simulink model "Control_System"  (R2018b)
settings: Solver=FixedStepAuto  StartTime=0.0  StopTime=10.0  FixedStep=global_time_step  RelTol=1e-3
values from neighbouring files (symbols this model uses):
  SRC_Ts = global_time_step    (= 0.001)    [Parameters.m]
  TFO_Ts = global_time_step    (= 0.001)    [Parameters.m]
undefined symbols (not defined in the file or in its folder): DiscIntNeverNeededParam, tyre_radius
libraries: simulink x2
settings Model: PauseTimes=1  Creator=univ4123  LastModifiedBy=univ4123
settings OptimizationCC: LifeSpan=inf
settings DebuggingCC: SFUnexpectedBacktrackingDiag=warning  SFNoUnconditionalDefaultTransitionDiag=warning
settings SFSimCC: SimUseLocalCustomCode=off
settings RTWCC: GenCodeOnly=on  RTWUseLocalCustomCode=off  Toolchain=MinGW64 | gmake (64-bit Windows)
settings CodeAppCC: StateflowObjectComments=on
settings GRTTargetCC: GeneratePreprocessorConditionals=Disable all
settings ConfigComp: CovMetricSettings=dw  CovHtmlReporting=on  CovSaveCumulativeToWorkspaceVar=on  CovSaveSingleToWorkspaceVar=on  CovExternalEMLEnable=off

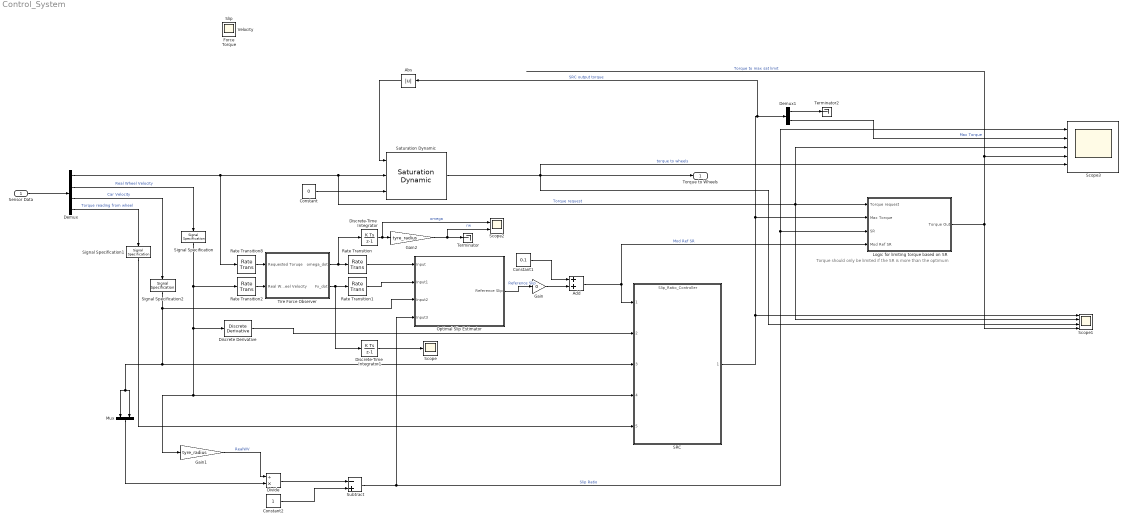
== system Control_System ==
  note: Torque should only be limited if the SR is more than the optimum
  Sensor Data : Inport
  Abs : Abs
  Add : Sum
  Constant : Constant  Value=0
  Constant1 : Constant  Value=0.1  SampleTime=SRC_Ts
  Constant2 : Constant  SampleTime=SRC_Ts
  Demux : Demux
  Demux1 : Demux  Outputs=2
  Discrete Derivative : simulink/Discrete/Discrete Derivative  gainval=1.0  ICPrevScaledInput=0.0  OutMin=[]  OutMax=[]  OutDataType=fixdt(1, 16)  OutScaling=2^-10  DoSatur=off
  Discrete-Time Integrator : DiscreteIntegrator  SampleTime=TFO_Ts  ICPrevOutput=DiscIntNeverNeededParam  ICPrevScaledInput=DiscIntNeverNeededParam
  Discrete-Time Integrator1 : DiscreteIntegrator  SampleTime=-1  ICPrevOutput=DiscIntNeverNeededParam  ICPrevScaledInput=DiscIntNeverNeededParam
  Divide : Product  Inputs=/*
  Gain : Gain  Gain=0
  Gain1 : Gain  Gain=tyre_radius
  Gain2 : Gain  Gain=tyre_radius
  Logic for limiting torque based on SR : Subsystem
  Mux : Mux  Inputs=2
  Optimal Slip Estimator : Subsystem
  Rate Transition : RateTransition  OutPortSampleTime=OSE_Ts
  Rate Transition1 : RateTransition  OutPortSampleTime=OSE_Ts
  Rate Transition2 : RateTransition  OutPortSampleTime=TFO_Ts
  Rate Transition8 : RateTransition  OutPortSampleTime=TFO_Ts
  SRC : ModelReference  ModelNameDialog=Slip_Ratio_Controller.slx  SimulationMode=Normal  ModelReferenceVersion=1.104
  Saturation Dynamic : simulink/Discontinuities/Saturation Dynamic  OutMin=[]  OutMax=[]  OutDataTypeStr=Inherit: Same as second input  OutDataType=fixdt(1, 16)  OutScaling=2^-10  DoSatur=off
  Scope : Scope
  Scope1 : Scope  NumInputPorts=4
  Scope2 : Scope  NumInputPorts=2
  Scope3 : Scope  NumInputPorts=5
  Signal Specification : SignalSpecification  Dimensions=[2 1]
  Signal Specification1 : SignalSpecification  Dimensions=1
  Signal Specification2 : SignalSpecification  Dimensions=1
  Subtract : Sum  Inputs=-+
  Terminator : Terminator
  Terminator2 : Terminator
  Tire Force Observer : Subsystem
  Torque to Wheels : Outport
  Force : Scope
  Slip : Scope
  Torque : Scope
  Velocity : Scope
  wires:
  Demux/1 -> Scope1/2, Scope3/3, Logic for limiting torque based on SR/1(Torque request), Saturation Dynamic/2, Rate Transition8/1  "Torque request"
  Saturation Dynamic/1 -> Scope1/3, Torque to Wheels/1, Scope3/5  "torque to wheels"
  Tire Force Observer/1(omega_dot) -> Discrete-Time Integrator/1, Rate Transition/1
  SRC/1 -> Abs/1, Demux1/1, Logic for limiting torque based on SR/2(Max Torque), Scope1/1  "SRC output torque"
  Constant/1 -> Saturation Dynamic/3
  Sensor Data/1 -> Demux/1
  Demux/2 -> Signal Specification/1  "Real Wheel Velocity"
  Demux/3 -> Signal Specification2/1  "Car Velocity"
  Rate Transition/1 -> Optimal Slip Estimator/1(Input)
  Tire Force Observer/2(Fx_dot) -> Discrete-Time Integrator1/1, Rate Transition1/1
  Gain/1 -> Add/2
  Constant1/1 -> Add/1
  Discrete-Time Integrator/1 -> Scope2/1, Gain2/1  "omega"
  Demux/4 -> Signal Specification1/1  "Torque reading from wheel"
  Rate Transition8/1 -> Tire Force Observer/1(Requested Toruqe)
  Rate Transition2/1 -> Tire Force Observer/2(Real Wheel Velocity)
  Rate Transition1/1 -> Optimal Slip Estimator/2(Input1)
  Signal Specification1/1 -> SRC/5
  Signal Specification2/1 -> Optimal Slip Estimator/3(Input2), Mux/1, Mux/2, SRC/3
  Logic for limiting torque based on SR/1(Torque Out) -> Scope3/4, Scope1/4  "Torque to max sat limit"
  Signal Specification/1 -> Rate Transition2/1, Gain1/1, SRC/4, Discrete Derivative/1
  Divide/1 -> Subtract/1
  Mux/1 -> Divide/2
  Gain1/1 -> Divide/1  "RealWV"
  Constant2/1 -> Subtract/2
  Add/1 -> Logic for limiting torque based on SR/4(Mod Ref SR), SRC/1  "Mod Ref SR"
  Optimal Slip Estimator/1(Reference Slip) -> Gain/1  "Reference Slip"
  Gain2/1 -> Scope2/2, Terminator/1  "rw"
  Discrete-Time Integrator1/1 -> Scope/1
  Discrete Derivative/1 -> SRC/2
  Subtract/1 -> Optimal Slip Estimator/4(Input3), Scope3/1, Logic for limiting torque based on SR/3(SR)  "Slip Ratio"
  Demux1/2 -> Scope3/2  "Max Torque"
  Demux1/1 -> Terminator2/1
  Abs/1 -> Saturation Dynamic/1

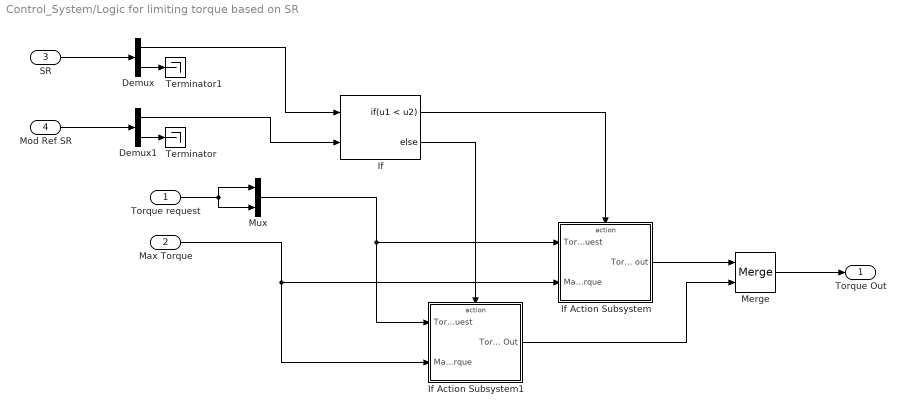
== system Control_System/Logic for limiting torque based on SR ==
  Torque request : Inport
  Max Torque : Inport  Port=2
  SR : Inport  Port=3
  Mod Ref SR : Inport  Port=4
  Demux : Demux  Outputs=2
  Demux1 : Demux  Outputs=2
  If : If  NumInputs=2  IfExpression=u1 < u2
  If Action Subsystem : Subsystem  TreatAsAtomicUnit=on
  If Action Subsystem1 : Subsystem  TreatAsAtomicUnit=on
  Merge : Merge
  Mux : Mux  Inputs=2
  Terminator : Terminator
  Terminator1 : Terminator
  Torque Out : Outport
  wires:
  SR/1 -> Demux/1
  Mod Ref SR/1 -> Demux1/1
  If/2 -> If Action Subsystem1/Action
  Mux/1 -> If Action Subsystem1/1(Torque Request), If Action Subsystem/1(Torque Request)
  Max Torque/1 -> If Action Subsystem1/2(Max Torque), If Action Subsystem/2(Max Torque)
  Merge/1 -> Torque Out/1
  If Action Subsystem/1(Torque out) -> Merge/1
  If Action Subsystem1/1(Torque Out) -> Merge/2
  Demux/1 -> If/1
  If/1 -> If Action Subsystem/Action
  Torque request/1 -> Mux/2, Mux/1
  Demux1/1 -> If/2
  Demux1/2 -> Terminator/1
  Demux/2 -> Terminator1/1

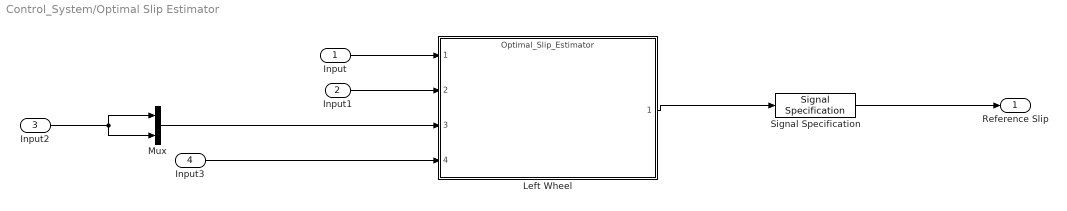
== system Control_System/Optimal Slip Estimator ==
  Input : Inport
  Input1 : Inport  Port=2
  Input2 : Inport  Port=3
  Input3 : Inport  Port=4
  Left Wheel : ModelReference  ModelNameDialog=Optimal_Slip_Estimator  SimulationMode=Normal  ModelReferenceVersion=1.13
  Mux : Mux  Inputs=2
  Signal Specification : SignalSpecification  Dimensions=[2 1]
  Reference Slip : Outport
  wires:
  Left Wheel/1 -> Signal Specification/1
  Signal Specification/1 -> Reference Slip/1
  Input/1 -> Left Wheel/1
  Input1/1 -> Left Wheel/2
  Input3/1 -> Left Wheel/4
  Mux/1 -> Left Wheel/3
  Input2/1 -> Mux/2, Mux/1

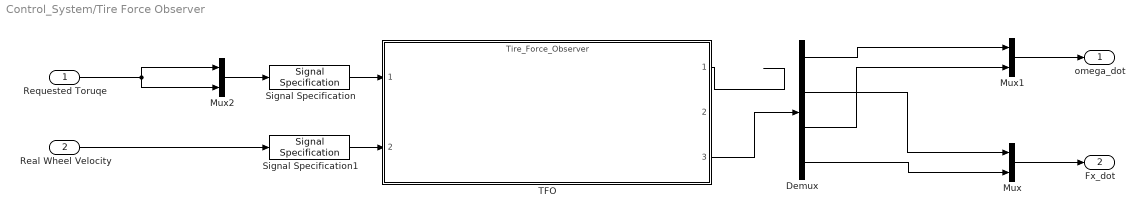
== system Control_System/Tire Force Observer ==
  Requested Toruqe : Inport
  Real Wheel Velocity : Inport  Port=2
  Demux : Demux
  Mux : Mux  Inputs=2
  Mux1 : Mux  Inputs=2
  Mux2 : Mux  Inputs=2
  Signal Specification : SignalSpecification  Dimensions=[2 1]
  Signal Specification1 : SignalSpecification  Dimensions=[2 1]
  TFO : ModelReference  ModelNameDialog=Tire_Force_Observer.slx  SimulationMode=Normal  ModelReferenceVersion=1.6
  omega_dot : Outport
  Fx_dot : Outport  Port=2
  wires:
  Requested Toruqe/1 -> Mux2/2, Mux2/1
  Real Wheel Velocity/1 -> Signal Specification1/1
  TFO/1 -> ?
  Mux1/1 -> omega_dot/1
  Demux/4 -> Mux/2
  Mux/1 -> Fx_dot/1
  Demux/2 -> Mux/1
  Demux/3 -> Mux1/2
  Demux/1 -> Mux1/1
  Mux2/1 -> Signal Specification/1
  Signal Specification/1 -> TFO/1
  Signal Specification1/1 -> TFO/2
  TFO/3 -> Demux/1

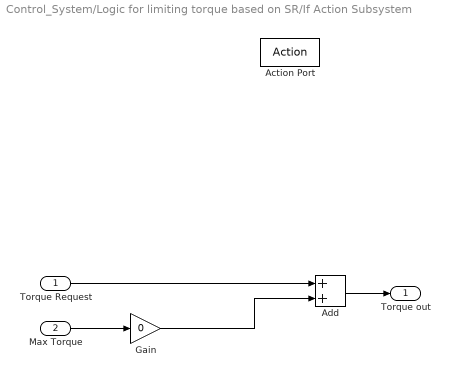
== system Control_System/Logic for limiting torque based on SR/If Action Subsystem ==
  Torque Request : Inport
  Max Torque : Inport  Port=2
  Action Port : ActionPort  ActionType=then
  Add : Sum
  Gain : Gain  Gain=0
  Torque out : Outport
  wires:
  Add/1 -> Torque out/1
  Gain/1 -> Add/2
  Max Torque/1 -> Gain/1
  Torque Request/1 -> Add/1

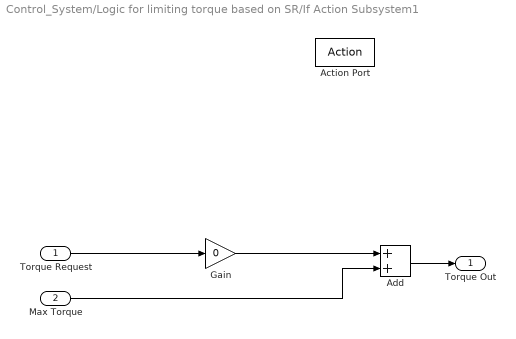
== system Control_System/Logic for limiting torque based on SR/If Action Subsystem1 ==
  Torque Request : Inport
  Max Torque : Inport  Port=2
  Action Port : ActionPort  ActionType=else
  Add : Sum
  Gain : Gain  Gain=0
  Torque Out : Outport
  wires:
  Gain/1 -> Add/1
  Add/1 -> Torque Out/1
  Torque Request/1 -> Gain/1
  Max Torque/1 -> Add/2
